simulink model "exp2_3_1"  (R2013a)
settings: Solver=ode45  StartTime=0.0  StopTime=400  RelTol=1e-3
settings Model: Creator=wyh716  LastModifiedBy=wyh716
settings DataIOCC: SignalLoggingSaveFormat=ModelDataLogs
settings DebuggingCC: MultiTaskDSMMsg=warning  MultiTaskCondExecSysMsg=none  StrictBusMsg=None
settings RTWCC: IncludeERTFirstTime=on
settings GRTTargetCC: CodeReplacementLibrary=None  CPPClassGenCompliant=on

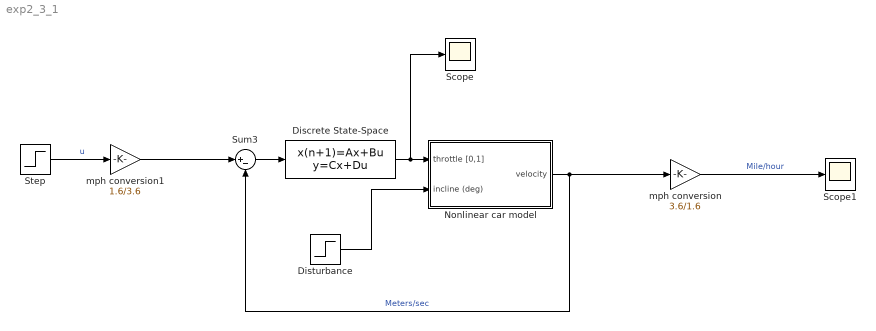
== system exp2_3_1 ==
  Discrete State-Space : DiscreteStateSpace  B=0.01  C=0.9094  D=1.15  X0=.2606  SampleTime=0.01
  Disturbance : Step  Time=100  After=0  SampleTime=0
  Nonlinear car model : Subsystem  mask{ca=1*1500, cf=1*1500/55/55, m=1500}
      mask prompts: ca "acceleration coeff"; cf "friction/aero coeff"; m "mass"
  Scope : Scope
  Scope1 : Scope
      settings: TimeRange=200  YMin=38.5  YMax=42.5
  Step : Step  Time=10  Before=60  After=65  SampleTime=0
  Sum3 : Sum  Inputs=|+-
  mph conversion : Gain  Gain=3.6/1.6  SaturateOnIntegerOverflow=on  OutDataTypeStr=Inherit: Same as input  ParamDataTypeStr=Inherit: Same as input
  mph conversion1 : Gain  Gain=1.6/3.6  SaturateOnIntegerOverflow=on  OutDataTypeStr=Inherit: Same as input  ParamDataTypeStr=Inherit: Same as input
  wires:
  mph conversion/1 -> Scope1/1  "Mile/hour"
  Nonlinear car model/1(velocity) -> Sum3/2, mph conversion/1  "Meters/sec"
  Step/1 -> mph conversion1/1  "u"
  mph conversion1/1 -> Sum3/1
  Disturbance/1 -> Nonlinear car model/2(incline (deg))
  Sum3/1 -> Discrete State-Space/1
  Discrete State-Space/1 -> Scope/1, Nonlinear car model/1(throttle [0,1])

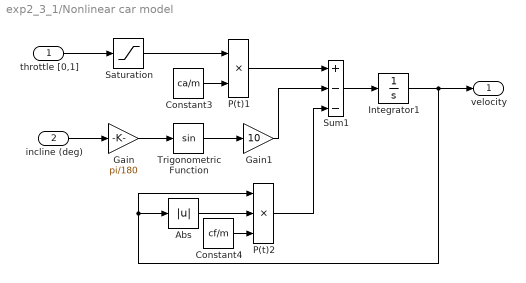
== system exp2_3_1/Nonlinear car model ==
  throttle [0,1] : Inport
  incline (deg) : Inport  Port=2
  Abs : Abs  SaturateOnIntegerOverflow=on
  Constant3 : Constant  Value=ca/m
  Constant4 : Constant  Value=cf/m
  Gain : Gain  Gain=pi/180  SaturateOnIntegerOverflow=on  OutDataTypeStr=Inherit: Same as input  ParamDataTypeStr=Inherit: Same as input
  Gain1 : Gain  Gain=10  SaturateOnIntegerOverflow=on  OutDataTypeStr=Inherit: Same as input  ParamDataTypeStr=Inherit: Same as input
  Integrator1 : Integrator  InitialCondition=26.67  UpperSaturationLimit=1  LowerSaturationLimit=0
  P(t)1 : Product  Inputs=**  SaturateOnIntegerOverflow=on  RndMeth=Zero  InputSameDT=on  OutDataTypeStr=Inherit: Same as first input
  P(t)2 : Product  Inputs=***  SaturateOnIntegerOverflow=on  RndMeth=Zero  InputSameDT=on  OutDataTypeStr=Inherit: Same as first input
  Saturation : Saturate  UpperLimit=3  LowerLimit=-1
  Sum1 : Sum  Inputs=+--  SaturateOnIntegerOverflow=on  InputSameDT=on  OutDataTypeStr=Inherit: Same as first input
  Trigonometric Function : Trigonometry
  velocity : Outport
  wires:
  Saturation/1 -> P(t)1/1
  Sum1/1 -> Integrator1/1
  Constant3/1 -> P(t)1/2
  P(t)1/1 -> Sum1/1
  Integrator1/1 -> Abs/1, P(t)2/1, velocity/1
  Constant4/1 -> P(t)2/3
  throttle [0,1]/1 -> Saturation/1
  incline (deg)/1 -> Gain/1
  P(t)2/1 -> Sum1/3
  Gain/1 -> Trigonometric Function/1
  Gain1/1 -> Sum1/2
  Trigonometric Function/1 -> Gain1/1
  Abs/1 -> P(t)2/2
